simulink model "Ohm_low"  (R2020a)
settings: Solver=VariableStepAuto  StartTime=0.0  StopTime=10.0  RelTol=1e-3
settings Model: Creator=Administrator  LastModifiedBy=Administrator

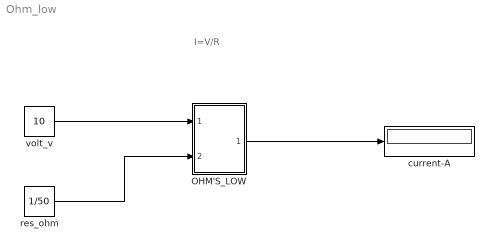
== system Ohm_low ==
  note: I=V/R
  OHM'S_LOW : Subsystem
  current-A : Display
  res_ohm : Constant  Value=1/50
  volt_v : Constant  Value=10
  wires:
  volt_v/1 -> OHM'S_LOW/1(voltage)
  res_ohm/1 -> OHM'S_LOW/2(1/res)
  OHM'S_LOW/1(current) -> current-A/1

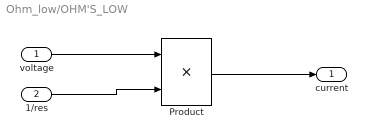
== system Ohm_low/OHM'S_LOW ==
  voltage : Inport
  1/res : Inport  Port=2
  Product : Product
  current : Outport
  wires:
  1/res/1 -> Product/2
  voltage/1 -> Product/1
  Product/1 -> current/1
